simulink model "chiller"  (R2021b)
settings: Solver=FixedStepAuto  StartTime=0.0  StopTime=200  RelTol=1e-3  AbsTol=1e-3  EnableMultiTasking=on
PreLoadFcn:
  | load r134aPropertyTables
  | 
  | % Refrigerant:
  | initial_pressure = 0.6; % MPa
  | initial_quality = 0.05;
  | 
  | % Environment:
  | environment_temperature = 293; % K
  | natural_convection_coefficient = 20; % W/m^2/K
  | 
  | % Controller:
  | target_temperature = 277; % K
  | temperature_delta = 2; % K
  | 
  | % Compressor:
  | commanded_mass_flow = 0.004; % kg/s
  | controller_time_constant = 20; % s
  | 
  | % Expansion valve:
  | min_throat_area = 0.1; % mm^2
  | max_throat_area = 1.5; % mm^2
  | min_throat_temperature = 270; % K
  | max_throat_temperature = 250; % K
  | 
  | % Heat exchangers:
  | condenser_length = 30; % m
  | evaporator_length = 30; % m
  | fin_area = 1; % m^2
  | fin_convection_coefficient = 150; % W/m^2/K
  | 
  | % Pipes:
  | pipe_diameter = 0.01; % m
  | pipe_thickness = 0.0005; % m
  | 
  | % Refrigerator compartment:
  | interior_surface_area = 4.5; % m^2
  | exterior_surface_area = 6; % m^2
  | foam_thickness = 0.03; % m
  | 
  | % Material properties:
  | copper_density = 8940; % kg/m^3
  | copper_specific_heat = 390; % J/kg/K
  | copper_conductivity = 400; % W/m/K
  | foam_conductivity = 0.03; % W/m/K
undefined symbols (not defined in the file): hx_length, initTemp, sh_sp, SHC5018sp, STC5018sp, swep_radius, TC5018sp
libraries: fl_lib x105, nesl_utility x33, slpidlib x5, SimscapeFluids_lib x1
(part 3 of 3)

== system chiller/Expansion Valve2/Cycle Sensor 3 ==
  Absolute Reference (2P) : fl_lib/Two-Phase Fluid/Elements/Absolute Reference (2P)
      settings: SourceProductBaseCode=SS
  Pressure & Internal Energy Sensor (2P) : fl_lib/Two-Phase Fluid/Sensors/Pressure & Internal Energy Sensor (2P)
      settings: SourceProductBaseCode=SS  InternalSimscapePortConfiguration="{\"Bottom\":[],\"Left\":[{\"id\":\"A\",\"label\":\"A\",\"type\":\"foundation.two_phase_fluid.two_phase_fluid\"}],\"Right\":[{\"id\":\"B\",\"label\":\"B\",\"type\":\"foundation.two_phase_fluid.two_phase_fluid\"},{\"id\":\"P\",\"label\":\"P\",\"type\":\"output\"},{\"id\":\"U\",\"label\":\"U\",\"type\":\"output\"}],\"Top\":[]}"
  Thermodynamic Properties Sensor (2P) : fl_lib/Two-Phase Fluid/Sensors/Thermodynamic Properties Sensor (2P)
      settings: SourceProductBaseCode=SS  InternalSimscapePortConfiguration="{\"Bottom\":[],\"Left\":[{\"id\":\"A\",\"label\":\"A\",\"type\":\"foundation.two_phase_fluid.two_phase_fluid\"}],\"Right\":[{\"id\":\"T\",\"label\":\"T\",\"type\":\"output\"},{\"id\":\"H\",\"label\":\"h\",\"type\":\"output\"},{\"id\":\"V\",\"label\":\"v\",\"type\":\"output\"},{\"id\":\"S\",\"label\":\"s\",\"type\":\"output\"}],\"Top\":[]}"
  Vapor Quality Sensor (2P) : fl_lib/Two-Phase Fluid/Sensors/Vapor Quality Sensor (2P)  vapor_fraction_spec=foundation.enum.vapor_fraction_spec.quality
      settings: SourceProductBaseCode=SS  InternalSimscapePortConfiguration="{\"Bottom\":[],\"Left\":[{\"id\":\"A\",\"label\":\"A\",\"type\":\"foundation.two_phase_fluid.two_phase_fluid\"}],\"Right\":[{\"id\":\"X\",\"label\":\"X\",\"type\":\"output\"}],\"Top\":[]}"
  A : PMIOPort  Side=Left
  connections:
  Thermodynamic Properties Sensor (2P)/LConn1 -- Vapor Quality Sensor (2P)/LConn1 -- A/RConn1 -- Pressure & Internal Energy Sensor (2P)/LConn1
  Absolute Reference (2P)/LConn1 -- Pressure & Internal Energy Sensor (2P)/RConn1

== system chiller/Expansion Valve2/Mass Flow Sensor ==
  Mass & Energy Flow Rate Sensor (2P) : fl_lib/Two-Phase Fluid/Sensors/Mass & Energy Flow Rate Sensor (2P)
      settings: SourceProductBaseCode=SS  InternalSimscapePortConfiguration="{\"Bottom\":[],\"Left\":[{\"id\":\"A\",\"label\":\"A\",\"type\":\"foundation.two_phase_fluid.two_phase_fluid\"}],\"Right\":[{\"id\":\"B\",\"label\":\"B\",\"type\":\"foundation.two_phase_fluid.two_phase_fluid\"},{\"id\":\"M\",\"label\":\"M\",\"type\":\"output\"},{\"id\":\"PHI\",\"label\":\"Phi\",\"type\":\"output\"}],\"Top\":[]}"
  PS-Simulink Converter : nesl_utility/PS-Simulink Converter  PhysicalDomain=network_engine_domain  SubClassName=ps_output  LeftPortType=input  RightPortType=output  PseudoPeriodic=off  Frequencies=[]  Unit=inherit  AffineConversion=off
      settings: SourceProductBaseCode=PW,SS
  B : PMIOPort  Side=Right
  A : PMIOPort  Port=2  Side=Left
  wires:
  PS-Simulink Converter/1 -> ?
  connections:
  Mass & Energy Flow Rate Sensor (2P)/LConn1 -- A/RConn1
  Mass & Energy Flow Rate Sensor (2P)/RConn1 -- B/RConn1
  PS-Simulink Converter/LConn1 -- Mass & Energy Flow Rate Sensor (2P)/RConn2
